simulink model "Input_Conversion"  (R2017b)
settings: configuration reference "Autosar_CodeGeneration" (kept outside this file)
settings Model: RequirementInfo={'linktype_rmi_url' 'http://md1hxhhc.ww004.siemens.net/polarion/' '@/project/ATRover/workitem?id=ATR-527' 'true' 'Polarion: ATR-527' '' } %GIDa_3f3a77ed_89ee_4fca_bcf7_4f28e7f20a28  DataDictionary=RoverDataDict.sldd  Creator=zwqe6u  LastModifiedBy=eh6qym
settings ConfigSetRef: DDName=RoverDataDict.sldd

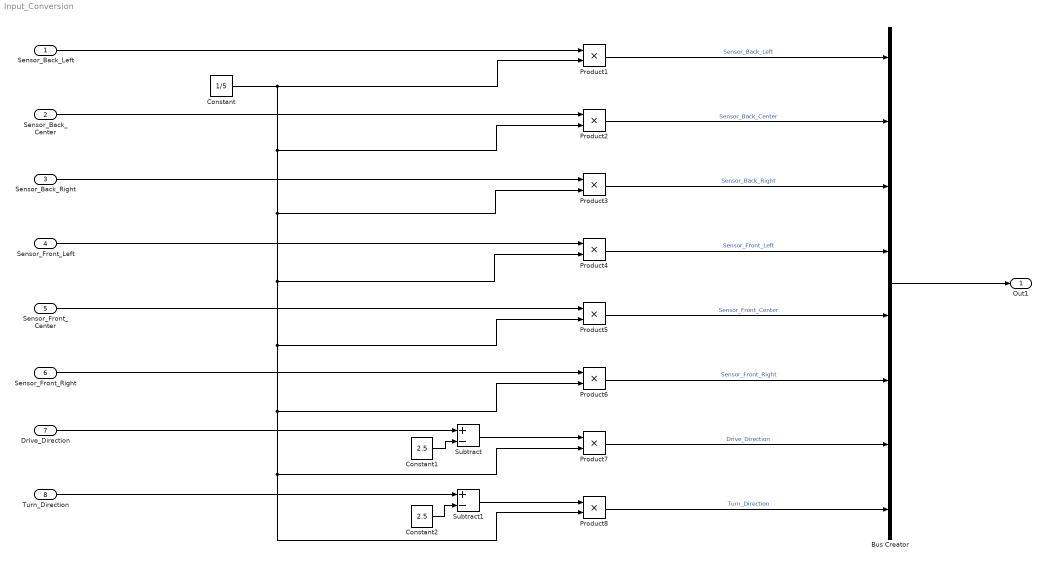
== system Input_Conversion ==
  Sensor_Back_Left : Inport  OutDataTypeStr=double  PortDimensions=1
  Sensor_Back_Center : Inport  Port=2  OutDataTypeStr=double  PortDimensions=1
  Sensor_Back_Right : Inport  Port=3  OutDataTypeStr=double  PortDimensions=1
  Sensor_Front_Left : Inport  Port=4  OutDataTypeStr=double  PortDimensions=1
  Sensor_Front_Center : Inport  Port=5  OutDataTypeStr=double  PortDimensions=1
  Sensor_Front_Right : Inport  Port=6  OutDataTypeStr=double  PortDimensions=1
  Drive_Direction : Inport  Port=7  OutDataTypeStr=double  PortDimensions=1
  Turn_Direction : Inport  Port=8  OutDataTypeStr=double  PortDimensions=1
  Bus Creator : BusCreator  Inputs=8
  Constant : Constant  Value=1/5
  Constant1 : Constant  Value=2.5
  Constant2 : Constant  Value=2.5
  Product1 : Product  OutDataTypeStr=Inherit: Inherit via back propagation
  Product{2..8} (7 alike) : Product
  Subtract : Sum  Inputs=+-
  Subtract1 : Sum  Inputs=+-
  Out1 : Outport  OutDataTypeStr=Bus: DAQ_In
  wires:
  Bus Creator/1 -> Out1/1
  Sensor_Back_Left/1 -> Product1/1
  Product1/1 -> Bus Creator/1  "Sensor_Back_Left"
  Sensor_Back_Center/1 -> Product2/1
  Product2/1 -> Bus Creator/2  "Sensor_Back_Center"
  Sensor_Back_Right/1 -> Product3/1
  Product3/1 -> Bus Creator/3  "Sensor_Back_Right"
  Sensor_Front_Left/1 -> Product4/1
  Product4/1 -> Bus Creator/4  "Sensor_Front_Left"
  Sensor_Front_Center/1 -> Product5/1
  Product5/1 -> Bus Creator/5  "Sensor_Front_Center"
  Sensor_Front_Right/1 -> Product6/1
  Product6/1 -> Bus Creator/6  "Sensor_Front_Right"
  Product7/1 -> Bus Creator/7  "Drive_Direction"
  Product8/1 -> Bus Creator/8  "Turn_Direction"
  Constant/1 -> Product5/2, Product7/2, Product8/2, Product6/2, Product4/2, Product3/2, Product2/2, Product1/2
  Subtract/1 -> Product7/1
  Drive_Direction/1 -> Subtract/1
  Subtract1/1 -> Product8/1
  Turn_Direction/1 -> Subtract1/1
  Constant1/1 -> Subtract/2
  Constant2/1 -> Subtract1/2
